simulink model "DDMR_ADRC_LSTM_RL"  (R2023b)
settings: Solver=ode4  StartTime=0.0  StopTime=31  FixedStep=0.01  RelTol=1e-5
libraries: simulink x2, deeplib x1, rllib x1
settings Model: Creator=Dell  LastModifiedBy=Dell
settings DebuggingCC: AlgebraicLoopMsg=none  SigSpecEnsureSampleTimeMsg=none

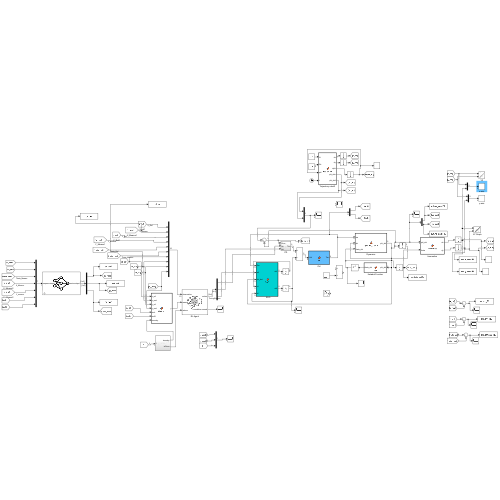
[thumbnail: Simulink's stored preview of the top-level diagram]
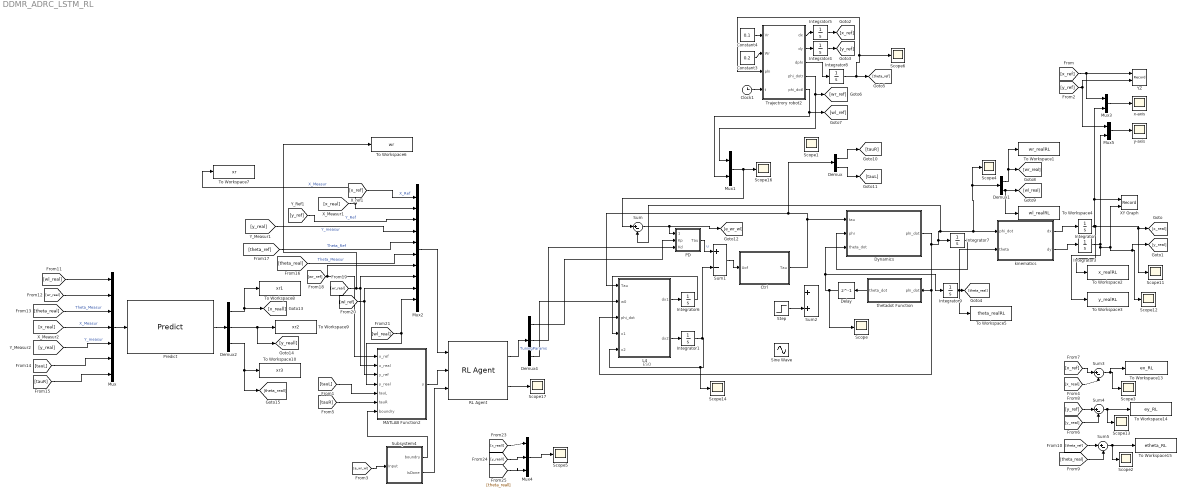
== system DDMR_ADRC_LSTM_RL ==
  note: ESO
  Clock1 : Clock
  Constant3 : Constant  Value=0.2
  Constant4 : Constant  Value=0.1
  Ctrl : MATLAB Function  TreatAsAtomicUnit=on
  Delay : Delay  DelayLength=1  InitialCondition=0
  Demux : Demux  Outputs=2
  Demux1 : Demux  Outputs=2
  Demux2 : Demux  Outputs=3
  Demux4 : Demux  Outputs=3
  Dynamics : MATLAB Function  TreatAsAtomicUnit=on
  Integrator{,3..5,8..9} (6 alike) : Integrator
  Integrator1 : Integrator  InitialCondition=[0;0]
  Integrator6 : Integrator  InitialCondition=[0;0]
  Integrator7 : Integrator  InitialCondition=[0;0]
  L4 : MATLAB Function  TreatAsAtomicUnit=on
  MATLAB Function2 : MATLAB Function  TreatAsAtomicUnit=on
  Mux : Mux  Inputs=7
  Mux1 : Mux  Inputs=2
  Mux2 : Mux  Inputs=10
  Mux3 : Mux  Inputs=2
  Mux4 : Mux  Inputs=3
  Mux5 : Mux  Inputs=2
  PD : Subsystem
  Predict : deeplib/Predict  Network=Network from MAT-file  NetworkFunction=squeezenet  NetworkFilePath=C:\Users\Dell\Desktop\RA\Mobile robot\trainedLSTMModel.mat  MiniBatchSize=128  InputDataFormats={'',''}  Predictions=on  Activations={}  ForceInterpretedSim=off  EnableDLNetwork=on
  RL Agent : rllib/RL Agent  Agent=agent  ExternalActionAsInput=off  ProvideLastAction=off  ProvideCumRwd=on  TreatAsDirectFeedthrough=on  UseStrictObservationDataTypes=off
  Scope{,1..6,11..14,16..17} (13 alike) : Scope
  Sine Wave : Sin  Amplitude=5  SampleTime=0
  Step : Step  Time=5  SampleTime=0
  Subsystem4 : Subsystem
  Sum{,3..5} (4 alike) : Sum  Inputs=|+-
  Sum1 : Sum  Inputs=+-
  Sum2 : Sum
  To Workspace1 : ToWorkspace  VariableName=wr_realRL  SaveFormat=Timeseries  SampleTime=-1
  To Workspace10 : ToWorkspace  VariableName=xr3  SaveFormat=Timeseries  SampleTime=-1
  To Workspace13 : ToWorkspace  VariableName=ex_RL  SaveFormat=Timeseries  SampleTime=-1
  To Workspace14 : ToWorkspace  VariableName=ey_RL  SaveFormat=Timeseries  SampleTime=-1
  To Workspace15 : ToWorkspace  VariableName=etheta_RL  SaveFormat=Timeseries  SampleTime=-1
  To Workspace2 : ToWorkspace  VariableName=x_realRL  SaveFormat=Timeseries  SampleTime=-1
  To Workspace3 : ToWorkspace  VariableName=y_realRL  SaveFormat=Timeseries  SampleTime=-1
  To Workspace4 : ToWorkspace  VariableName=wl_realRL  SaveFormat=Timeseries  SampleTime=-1
  To Workspace5 : ToWorkspace  VariableName=theta_realRL  SaveFormat=Timeseries  SampleTime=-1
  To Workspace6 : ToWorkspace  VariableName=wr  SaveFormat=Timeseries  SampleTime=-1
  To Workspace7 : ToWorkspace  VariableName=xr  SaveFormat=Timeseries  SampleTime=-1
  To Workspace8 : ToWorkspace  VariableName=xr1  SaveFormat=Timeseries  SampleTime=-1
  To Workspace9 : ToWorkspace  VariableName=xr2  SaveFormat=Timeseries  SampleTime=-1
  Trajectrory robot2 : MATLAB Function  TreatAsAtomicUnit=on
  XY Graph : Record  FileSettingsInternal="{\"entries\":[{\"content\":{\"excelSettings\":{\"content\":{},\"type\":\"Streamout.ExcelSettings\"}},\"type\":\"Streamout.FileSettingStorage\",\"uuid\":\"\"}],\"packageUris\":[\"http:\\/\\/schema.mathworks.com\\/mf0\\/streamout_blocks\\/R2020a\"],\"version\":\"1.0\"}"  Layout=[1 1]  SignalsInternal="{\"entries\":[{\"content\":{\"signals\":[{\"content\":{\"blockPath\":[],\"dimensions\":[1],\"domain\":\"\",\"lineColor\":\"#a2142f\",\"plots\":[ 1 ],\"port\":1,\"sid\":[\"\"],\"signalID\":1,\"signalName\":\"Integrator\"},\"type\":\"RecordBlkView.Signal\",\"uuid\":\"\"},{\"content\":{\"blockPath\":[],\"dimensions\":[1],\"domain\":\"\",\"lineColor\":\"#139fff\",\"plots\":[ 1 ],\"port\":2,\"sid\":[\"\"],\"signalID\":2,\"signalName\":\"Integrator3\"},\"type\":\"RecordBlkView.Signal\",\"uuid\":\"\"}]},\"type\":\"RecordBlkView.InputSignals\",\"uuid\":\"\"}],\"packageUris\":[\"http:\\/\\/schema.mathworks.com\\/mf0\\/streamout_blocks\\/R2020a\"],\"version\":\"1.0\"}"  VisualizationBindings="{\"xyplotplugin\":{\"info\":[{\"series\":[{\"bindingParametersList\":[{\"parameter\":\"X-Axis\",\"signalID\":1,\"signalName\":\"Integrator\"},{\"parameter\":\"Y-Axis\",\"signalID\":2,\"signalName\":\"Integrator3\"}],\"seriesID\":0}],\"subplotID\":1}]}}"  CompatibilityTag=XY
  YZ : Record  FileSettingsInternal="{\"entries\":[{\"content\":{\"excelSettings\":{\"content\":{},\"type\":\"Streamout.ExcelSettings\"}},\"type\":\"Streamout.FileSettingStorage\",\"uuid\":\"\"}],\"packageUris\":[\"http:\\/\\/schema.mathworks.com\\/mf0\\/streamout_blocks\\/R2020a\"],\"version\":\"1.0\"}"  Layout=[1 1]  SignalsInternal="{\"entries\":[{\"content\":{\"signals\":[{\"content\":{\"blockPath\":[],\"dimensions\":[1],\"domain\":\"\",\"lineColor\":\"#a2142f\",\"plots\":[ 1 ],\"port\":1,\"sid\":[\"\"],\"signalID\":1,\"signalName\":\"From\"},\"type\":\"RecordBlkView.Signal\",\"uuid\":\"\"},{\"content\":{\"blockPath\":[],\"dimensions\":[1],\"domain\":\"\",\"lineColor\":\"#139fff\",\"plots\":[ 1 ],\"port\":2,\"sid\":[\"\"],\"signalID\":2,\"signalName\":\"From2\"},\"type\":\"RecordBlkView.Signal\",\"uuid\":\"\"}]},\"type\":\"RecordBlkView.InputSignals\",\"uuid\":\"\"}],\"packageUris\":[\"http:\\/\\/schema.mathworks.com\\/mf0\\/streamout_blocks\\/R2020a\"],\"version\":\"1.0\"}"  VisualizationBindings="{\"xyplotplugin\":{\"info\":[{\"series\":[{\"bindingParametersList\":[{\"parameter\":\"X-Axis\",\"signalID\":1,\"signalName\":\"From\"},{\"parameter\":\"Y-Axis\",\"signalID\":2,\"signalName\":\"From2\"}],\"seriesID\":0}],\"subplotID\":1}]}}"  CompatibilityTag=XY  st=-1
  kinematics : MATLAB Function  TreatAsAtomicUnit=on
  thetadot Function : MATLAB Function  TreatAsAtomicUnit=on
  x-axis : Scope
  y-axis : Scope
  wires:
  [tauR] -> MATLAB Function2/6(tauR)
  MATLAB Function2/1(y) -> RL Agent/2
  [tauL] -> MATLAB Function2/5(tauL)
  Subsystem4/1(boundry) -> MATLAB Function2/7(boundry)
  Subsystem4/2(IsDone) -> RL Agent/3
  RL Agent/2 -> Scope17/1
  RL Agent/1 -> Demux4/1  "TuningParams"
  [theta_real] -> Mux2/6  "Theta_Measur"
  [wl_ref] -> MATLAB Function2/3(y_ref), Mux2/9
  [x_real] -> To Workspace7/1, Mux2/2  "X_Measur"
  [wl_real] -> Mux2/10, MATLAB Function2/4(y_real)
  [y_real] -> Mux2/4  "Y_measur"
  [y_ref] -> Mux2/3  "Y_Ref"
  [theta_ref] -> Mux2/5  "Theta_Ref"
  [wr_ref] -> MATLAB Function2/1(x_ref), Mux2/7
  [wr_real] -> To Workspace6/1, MATLAB Function2/2(x_real), Mux2/8
  [x_ref] -> Mux2/1  "X_Ref"
  [x_ref] -> Mux3/1, YZ/1
  Demux1/2 -> To Workspace4/1, [wl_real]
  [y_ref] -> Mux5/1, YZ/2
  Demux/2 -> [tauL]
  Trajectrory robot2/4(phi_dotr) -> [wr_ref], Mux1/1
  L4/2(dx2) -> Integrator1/1
  Integrator4/1 -> [y_ref]
  Integrator7/1 -> Dynamics/2(phi)
  Integrator3/1 -> Scope12/1, [y_real], XY Graph/2, To Workspace3/1, Mux5/2
  L4/1(dx1) -> Integrator6/1
  thetadot Function/1(theta_dot) -> Delay/1
  PD/1(Tau) -> Sum1/1  "u"
  Mux5/1 -> y-axis/1
  Integrator/1 -> [x_real], Scope11/1, To Workspace2/1, XY Graph/1, Mux3/2
  kinematics/2(dy) -> Integrator3/1
  Integrator6/1 -> L4/4(x1)
  Demux/1 -> [tauR]
  Trajectrory robot2/5(phi_dotl) -> [wl_ref], Mux1/2
  Constant4/1 -> Trajectrory robot2/1(Vr)
  Mux1/1 -> Scope16/1, Sum/1
  Trajectrory robot2/2(dy) -> Integrator4/1
  Trajectrory robot2/3(dphi) -> Integrator8/1
  Sum/1 -> [e_wr_wl], PD/1(Error)
  Clock1/1 -> Trajectrory robot2/4(t)
  Demux4/3 -> L4/2(w0)
  Integrator8/1 -> [theta_ref], Trajectrory robot2/3(phi), Scope6/1
  Sum1/1 -> Ctrl/1(Uof)
  Constant3/1 -> Trajectrory robot2/2(Wr)
  kinematics/1(dx) -> Integrator/1
  Integrator1/1 -> Sum1/2, Scope14/1, L4/5(x2)
  Trajectrory robot2/1(dx) -> Integrator5/1
  Delay/1 -> Scope/1, Dynamics/3(theta_dot), Integrator9/1
  Dynamics/1(phi_dot) -> L4/3(phi_dot), thetadot Function/1(phi_dot), Sum/2, Scope4/1, Demux1/1, kinematics/1(phi_dot), Integrator7/1
  Demux1/1 -> To Workspace1/1, [wr_real]
  Mux3/1 -> x-axis/1
  Integrator5/1 -> [x_ref]
  Demux4/1 -> PD/2(Kp)
  Demux4/2 -> PD/3(Kd)
  [e_wr_wl] -> Subsystem4/1(Input)
  Integrator9/1 -> To Workspace5/1, kinematics/2(theta), [theta_real]
  [x_ref] -> Sum3/1
  [y_ref] -> Sum4/1
  Sum3/1 -> To Workspace13/1, Scope3/1
  Sum4/1 -> Scope13/1, To Workspace14/1
  [x_real] -> Sum3/2
  [y_real] -> Sum4/2
  Step/1 -> Sum2/2
  Sum5/1 -> Scope2/1, To Workspace15/1
  [theta_real] -> Sum5/2
  [theta_ref] -> Sum5/1
  Mux2/1 -> RL Agent/1
  [wl_real] -> Mux/1
  [tauL] -> Mux/6
  [theta_real] -> Mux/3  "Theta_Measur"
  [y_real] -> Mux/5  "Y_measur"
  [tauR] -> Mux/7
  [x_real] -> Mux/4  "X_Measur"
  [wr_real] -> Mux/2
  Mux/1 -> Predict/1
  Predict/1 -> Demux2/1
  Demux2/3 -> [theta_reall], To Workspace10/1
  Demux2/2 -> [y_reall], To Workspace9/1
  Demux2/1 -> [x_reall], To Workspace8/1
  [x_reall] -> Mux4/1
  [y_reall] -> Mux4/2
  [theta_reall] -> Mux4/3
  Mux4/1 -> Scope5/1
  Ctrl/1(Tau) -> Demux/1, L4/1(Tau), Dynamics/1(tau)

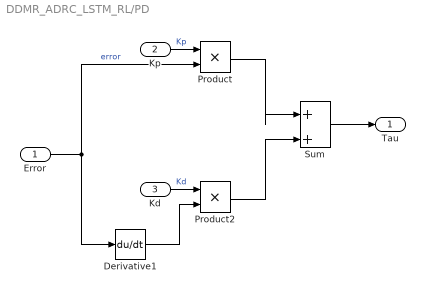
== system DDMR_ADRC_LSTM_RL/PD ==
  Error : Inport
  Kp : Inport  Port=2
  Kd : Inport  Port=3
  Derivative1 : Derivative
  Product : Product
  Product2 : Product
  Sum : Sum  Inputs=|++
  Tau : Outport
  wires:
  Derivative1/1 -> Product2/2
  Sum/1 -> Tau/1
  Product/1 -> Sum/1
  Error/1 -> Derivative1/1, Product/2  "error"
  Kd/1 -> Product2/1  "Kd"
  Kp/1 -> Product/1  "Kp"
  Product2/1 -> Sum/2

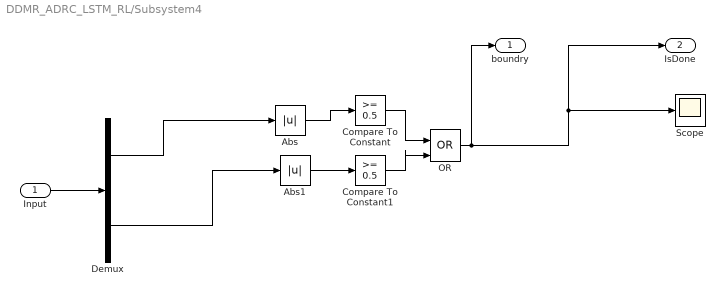
== system DDMR_ADRC_LSTM_RL/Subsystem4 ==
  Input : Inport
  Abs : Abs  SaturateOnIntegerOverflow=off
  Abs1 : Abs  SaturateOnIntegerOverflow=off
  Compare To Constant : simulink/Logic and Bit Operations/Compare To Constant  relop=>=  const=0.5  OutDataTypeStr=boolean
  Compare To Constant1 : simulink/Logic and Bit Operations/Compare To Constant  relop=>=  const=0.5  OutDataTypeStr=boolean
  Demux : Demux  Outputs=2
  OR : Logic  Operator=OR  IconShape=distinctive  AllPortsSameDT=off  OutDataTypeStr=boolean
  Scope : Scope
  boundry : Outport
  IsDone : Outport  Port=2
  wires:
  Input/1 -> Demux/1
  Demux/2 -> Abs1/1
  Demux/1 -> Abs/1
  Abs1/1 -> Compare To Constant1/1
  Abs/1 -> Compare To Constant/1
  Compare To Constant/1 -> OR/1
  OR/1 -> boundry/1, Scope/1, IsDone/1
  Compare To Constant1/1 -> OR/2

== matlab function DDMR_ADRC_LSTM_RL/thetadot Function ==
  data: phi_dot input; theta_dot output
function theta_dot = fcn(phi_dot)
L=0.24;
R=0.095;
theta_dot = 0;
phi_dotr = phi_dot(1);
phi_dotl = phi_dot(2);

w= (R .* (phi_dotr - phi_dotl))./ L;

theta_dot = w;

== matlab function DDMR_ADRC_LSTM_RL/Dynamics ==
  data: phi_dot output; tau input; phi input; theta_dot input
function phi_dot   = Dynamic_Model(tau, phi, theta_dot)
L=0.24;
R=0.095; %distnace between center and 1 wheel not 2 wheels distance
mc= 17;
mw= 0.5;
m= mc+(2*mw); %total mass of the robot
Ic=0.537;
Iw=0.0023;
Im=0.0011;
d=0.05;
I= Ic + (mc*(d^2)) + (2*mw*(L^2)) + (2*Im);

M11= Iw + ( ((R^2)/(4*(L^2))) * ((m*(L^2))+I) );
M12= ((R^2)/(4*(L^2))) * ((m*(L^2))-I);
M21= M12;
M22= M11;
M = [M11, M12; M21, M22];



V11= 0;
V12= ((R^2)/(4*L)) .* (mc*d.*theta_dot);
V21=-V12;
V22=0;
V = [V11, V12; V21, V22];

invM = inv(M);
phi_dot = invM * (tau - (V * phi));

== matlab function DDMR_ADRC_LSTM_RL/kinematics ==
  data: phi_dot input; dx output; dy output; theta input
function [dx, dy] = kinematics(phi_dot, theta)

R=0.095;

phi_dotr = phi_dot(1);
phi_dotl = phi_dot(2);
v= (R .* (phi_dotr + phi_dotl))/ 2;


dx =  v .* cos(theta);
dy =  v .* sin(theta);

== matlab function DDMR_ADRC_LSTM_RL/Ctrl ==
  data: Uof input; Tau output
function Tau = ctrl(Uof)
L=0.24;
R=0.095;
mc= 17;
mw= 0.5;
m= mc+(2*mw); %total mass of the robot
Ic=0.537;
Iw=0.0023;
Im=0.0011;
d=0.05;
I= Ic + (mc*(d^2)) + (2*mw*(L^2)) + (2*Im);

M11= Iw + ( ((R^2)/(4*(L^2))) * ((m*(L^2))+I) );
M12= ((R^2)/(4*(L^2))) * ((m*(L^2))-I);
M21= M12;
M22= M11;
M=[M11 M12;
    M21 M22];

Tau=M*Uof;
end

== matlab function DDMR_ADRC_LSTM_RL/L4 ==
  data: dx1 output; dx2 output; Tau input; w0 input; phi_dot input; x1 input; x2 input
function [dx1, dx2]=ESO(Tau,w0,phi_dot, x1,x2)
%R= 0.072;
%L= 0.21; %distnace between center and 1 wheel not 2 wheels distance
%mc= 20.1;
%mw= 0.15;
%m= 20.1+(2*0.15); %total mass of the robot

%Ic=0.1;
%Iw=0.001;
%Im=0.001;
%d=0.152;
%I= Ic + (mc*(d^2)) + (2*mw*(L^2)) + (2*Im);

L=0.24;
R=0.095;
mc= 17;
mw= 0.5;
m= mc+(2*mw); %total mass of the robot
Ic=0.537;
Iw=0.0023;
Im=0.0011;
d=0.05;
I= Ic + (mc*(d^2)) + (2*mw*(L^2)) + (2*Im);


M11= Iw + ( ((R^2)/(4*(L^2))) * ((m*(L^2))+I) );
M12= ((R^2)/(4*(L^2))) * ((m*(L^2))-I);
M21= M12;
M22= M11;
M=[M11 M12;
    M21 M22];




invM=inv(M);
% l1, l2, l3 ARE THE OBSERVER GAINS IN ESO calcualated using w0
L1=2*w0;   
L2=1*w0^2;

e = x1-phi_dot;

dx1=x2+(invM*Tau)-(L1.*e);
dx2= -(L2.*e);

== matlab function DDMR_ADRC_LSTM_RL/Trajectrory robot2 ==
  data: Vr input; Wr input; phi input; t input; dx output; dy output; dphi output; phi_dotr output; phi_dotl output
function [dx, dy, dphi, phi_dotr, phi_dotl] = desiredtraj(Vr, Wr, phi, t)
    d = 0.007; % Distance from center of rotation to the point of interest (if applicable)
    dx = cos(phi) * Vr + d * sin(phi) * Wr;
    dy = sin(phi) * Vr - d * cos(phi) * Wr;
    dphi = Wr;
    L=0.24;
    R=0.095;

    phi_dotr = (2 * Vr + Wr * L) ./ (2 * R);
    phi_dotl = (2 * Vr - Wr * L) ./ (2 * R);
    

end

== matlab function DDMR_ADRC_LSTM_RL/MATLAB Function2 ==
  data: x_ref input; y output; x_real input; y_ref input; y_real input; tauL input; tauR input; boundry input
function y = reward(x_ref, x_real,y_ref, y_real, tauL , tauR, boundry)
    % Position error (scaled)
    e_x = x_ref - x_real;
    
    e_y = y_ref - y_real;
    e= sqrt((e_x)^2 + (e_y)^2);
    % Torque penalty (scaled)
    %torq = (tauL^2 + tauR^2); 
    torq = abs(tauL) + abs(tauR);

    % Total reward: penalties + positive rewards
    y = - (0.001 *e) -(0.002 * torq) - 1*boundry ;

end
